simulink model "MPC_Ques1_Tube"  (R2024b)
settings: Solver=VariableStepAuto  StartTime=0.0  StopTime=30  RelTol=1e-3
libraries: mpclib x1, slpidlib x1
settings Model: Creator=Reza Shahriari  LastModifiedBy=Reza Shahriari

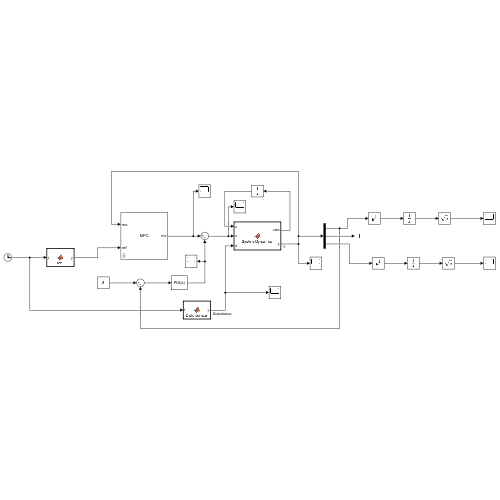
[thumbnail: Simulink's stored preview of the top-level diagram]
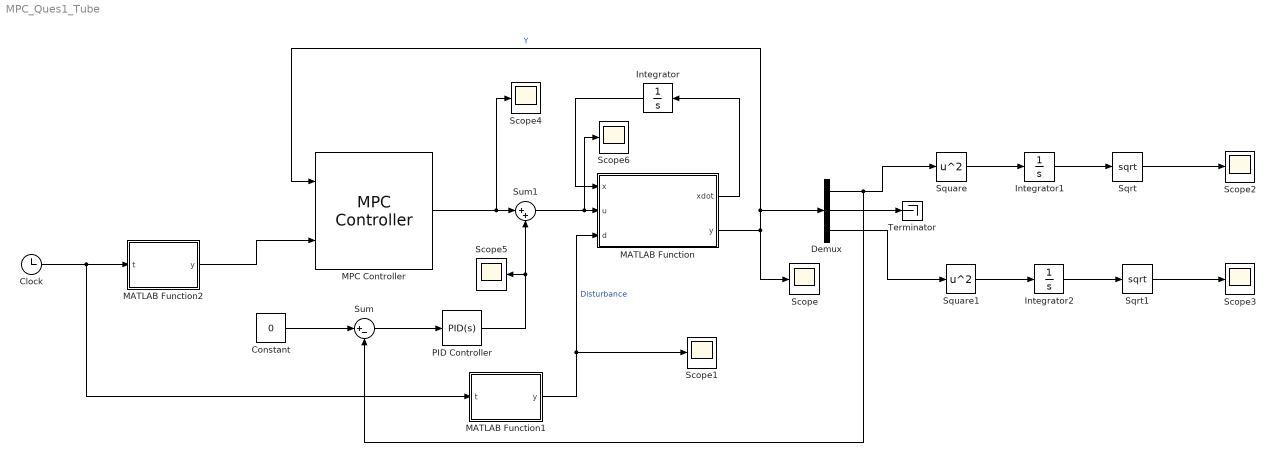
== system MPC_Ques1_Tube ==
  Clock : Clock
  Constant : Constant  Value=0
  Demux : Demux  Outputs=3
  Integrator : Integrator  InitialCondition=[0;0;0;0]
  Integrator1 : Integrator
  Integrator2 : Integrator
  MATLAB Function : MATLAB Function  TreatAsAtomicUnit=on
  MATLAB Function1 : MATLAB Function  TreatAsAtomicUnit=on
  MATLAB Function2 : MATLAB Function  TreatAsAtomicUnit=on
  MPC Controller : mpclib/MPC Controller  SCDEnableBlockLinearizationSpecification=on  mpcobj=mpc1  is_multiple=0  enable_value=0  return_u0=off  updateMPCinCallerWorkspace=on  md_inport=off  mv_inport=off  uref_inport=off  return_cost=off  return_mvseq=off  return_qpstatus=off  return_xseq=off  return_state=off  return_ovseq=off  state_inport=off  umin_inport=off  umax_inport=off  ymin_inport=off  ymax_inport=off  cc_inport=off  ywt_inport=off  uwt_inport=off  duwt_inport=off  rhoeps_inport=off  pm_inport=off  MaximumP=10  HorizonChoice=FixedHorizon  n_ts=0.01  n_p=100  n_mv=1  n_md=0  n_ud=0  n_mo=3  n_uo=0  BlockDataType=double  SampleTimeInherited=off  switch_inport=off
  PID Controller : slpidlib/PID Controller  Controller=PID  Form=Parallel  TimeDomain=Continuous-time  UseExternalTs=off  SampleTime=-1  IntegratorMethod=Forward Euler  FilterMethod=Forward Euler  ControllerParametersSource=internal  P=9680201.90683325  I=65547182.3865471  UseKiTs=off  D=353875.473741851  UseExternalDerivativeSource=off  N=1532.9863845951  UseFilter=on  TunerSelectOption=Transfer Function Based (PID Tuner App)  InitialConditionSource=internal  InitialConditionForIntegrator=0  InitialConditionForFilter=0  DifferentiatorICPrevScaledInput=0  ExternalReset=none  TrackingMode=off  Kt=1  LimitOutput=off  SatLimitsSource=internal  UpperSaturationLimit=inf  LowerSaturationLimit=-inf  LinearizeAsGain=on  AntiWindupMode=none  Kb=1  LimitIntegrator=off  UpperIntegratorSaturationLimit=inf  LowerIntegratorSaturationLimit=-inf  POutMin=[]  POutMax=[]  IOutMin=[]  IOutMax=[]  DOutMin=[]  DOutMax=[]  NOutMin=[]  NOutMax=[]  SumOutMin=[]  SumOutMax=[]  SaturationOutMin=[]  SaturationOutMax=[]  PParamMin=[]  PParamMax=[]  IParamMin=[]  IParamMax=[]  DParamMin=[]  DParamMax=[]  NParamMin=[]  NParamMax=[]  KbParamMin=[]  KbParamMax=[]  KtParamMin=[]  KtParamMax=[]  KbOutMin=[]  KbOutMax=[]  KtOutMin=[]  KtOutMax=[]  IntegratorOutMin=[]  IntegratorOutMax=[]  FilterOutMin=[]  FilterOutMax=[]  SumI1OutMin=[]  SumI1OutMax=[]  SumI2OutMin=[]  SumI2OutMax=[]  SumI3OutMin=[]  SumI3OutMax=[]  SumI4OutMin=[]  SumI4OutMax=[]  SumDOutMin=[]  SumDOutMax=[]  DifferentiatorOutMin=[]  DifferentiatorOutMax=[]  FilterDiffOutCoefMin=[]  FilterDiffOutCoefMax=[]  ReciprocalOutMin=[]  ReciprocalOutMax=[]  SumDenOutMin=[]  SumDenOutMax=[]  SumNumOutMin=[]  SumNumOutMax=[]  DivideOutMin=[]  DivideOutMax=[]  UdiffTsProdOutMin=[]  UdiffTsProdOutMax=[]  NTsProdOutMin=[]  NTsProdOutMax=[]  UintegralTsProdOutMin=[]  UintegralTsProdOutMax=[]  UngainTsProdOutMin=[]  UngainTsProdOutMax=[]  ClampingZeroOutDataTypeStr=Inherit: Inherit via back propagation  ClampingZeroOutMin=[]  ClampingZeroOutMax=[]  FilterDenConstantOutDataTypeStr=Inherit: Inherit via back propagation  FilterDenConstantOutMin=[]  FilterDenConstantOutMax=[]  PCopyOutDataTypeStr=Inherit: Inherit via back propagation  PCopyOutMin=[]  PCopyOutMax=[]  NCopyOutDataTypeStr=Inherit: Inherit via back propagation  NCopyOutMin=[]  NCopyOutMax=[]  IntegratorContinuousStateAttributes=''  IntegratorStateMustResolveToSignalObject=off  IntegratorRTWStateStorageClass=Auto  FilterContinuousStateAttributes=''  FilterStateMustResolveToSignalObject=off  FilterRTWStateStorageClass=Auto  ParallelPVariant=InternalParameters  IdealPVariant=Disabled  IVariant=InternalParameters  DVariant=InternalParameters  IntegratorVariant=Continuous  SatVariant=Disabled  AWVariant=Passthrough  PCopyVariant=Disabled  TRVariant=Disabled  FdbkBlocksVariant=Forward  IdealPFdbkVariant=Disabled  SatFdbkVariant=Disabled  DerivativeFilterVariant=ContFilter  NVariant=InternalParameters  NCopyVariant=Disabled  FilterICVariant=InternalICsFilter  IntegratorICVariant=InternalICs  ExternalResetVariant=Disabled  TRSumVariant=Passthrough  SumFdbkVariant=Disabled  SumVariant=Sum_PID  TsampFilterVariant=InternalTs  TsampNgainVariant=Passthrough  TsampIntegralVariant=Disabled_SignalSpec  ExternalSaturationOutDataTypeStr=Inherit: Same as second input  DerivativeSourceVariant=ErrorSignal  PreIntVariant=InternalPreInt
  Scope{,1..6} (7 alike) : Scope
  Sqrt : Sqrt
  Sqrt1 : Sqrt
  Square : Math  Operator=square
  Square1 : Math  Operator=square
  Sum : Sum  Inputs=|+-
  Sum1 : Sum  Inputs=|++
  Terminator : Terminator
  wires:
  Square/1 -> Integrator1/1
  MATLAB Function/2(y) -> MPC Controller/1, Demux/1, Scope/1  "Y"
  MATLAB Function1/1(y) -> MATLAB Function/3(d), Scope1/1  "Disturbance"
  Demux/2 -> Terminator/1
  Demux/1 -> Sum/2, Square/1
  Demux/3 -> Square1/1
  Integrator2/1 -> Sqrt1/1
  Square1/1 -> Integrator2/1
  Clock/1 -> MATLAB Function1/1(t), MATLAB Function2/1(t)
  Sqrt1/1 -> Scope3/1
  Sqrt/1 -> Scope2/1
  Integrator/1 -> MATLAB Function/1(x)
  Integrator1/1 -> Sqrt/1
  MATLAB Function/1(xdot) -> Integrator/1
  Sum/1 -> PID Controller/1
  Constant/1 -> Sum/1
  MPC Controller/1 -> Scope4/1, Sum1/1
  PID Controller/1 -> Sum1/2, Scope5/1
  Sum1/1 -> Scope6/1, MATLAB Function/2(u)
  MATLAB Function2/1(y) -> MPC Controller/2

== matlab function MPC_Ques1_Tube/MATLAB Function1 ==
  data: t input; y output
function y = Disturbance(t)

if t>=4 & t<5 
    y = t-4;
elseif t>=5 & t<7
    y = 1;
elseif t>=7 & t<8
    y = -t+8;
else 
    y = 0;
end

== matlab function MPC_Ques1_Tube/MATLAB Function ==
  data: x input; xdot output; u input; y output; d input
function [xdot,y]= SystemDynamics(x,u,d)

% Parameter Definition
Ms = 2500;
Mu = 320;
ks = 80000;
ku = 500000;
cs = 350;
cu = 15020;

A = [0 1 0 0;
     0 -cs/Ms -ks/Ms cs/Ms;
     0 1 0 -1;
     -ku/Mu cs/Mu (ks+ku)/Mu -(cs+cu)/Mu];
     
B = [0; 1/Ms; 0; -1/Mu];  % Input matrix

C = [1 0 0 0; 0 1 0 0; 0 0 1 0];


Diss = [0; cs*cu/(Ms*Mu); -cu/Mu; (cu/Mu)*(ku*cu-cs*Mu-cu*Mu)];

xdot = A*x + B*u + Diss*d;
y = C*x;

== matlab function MPC_Ques1_Tube/MATLAB Function2 ==
  data: y output; t input
function y = fcn(t)

y = [0;0;0];
